simulink model "Non_isolated_SEPIC"  (R2021a)
settings: Solver=VariableStepAuto  StartTime=0.0  StopTime=0.1  RelTol=1e-3
libraries: spsSeriesRLCBranchLib x8, spsCurrentMeasurementLib x3, spsVoltageMeasurementLib x2, spsDiodeLib x1, spsMosfetLib x1, spsDCVoltageSourceLib x1, spspowerguiLib x1
settings Model: Creator=EREN-PC  LastModifiedBy=EREN-PC

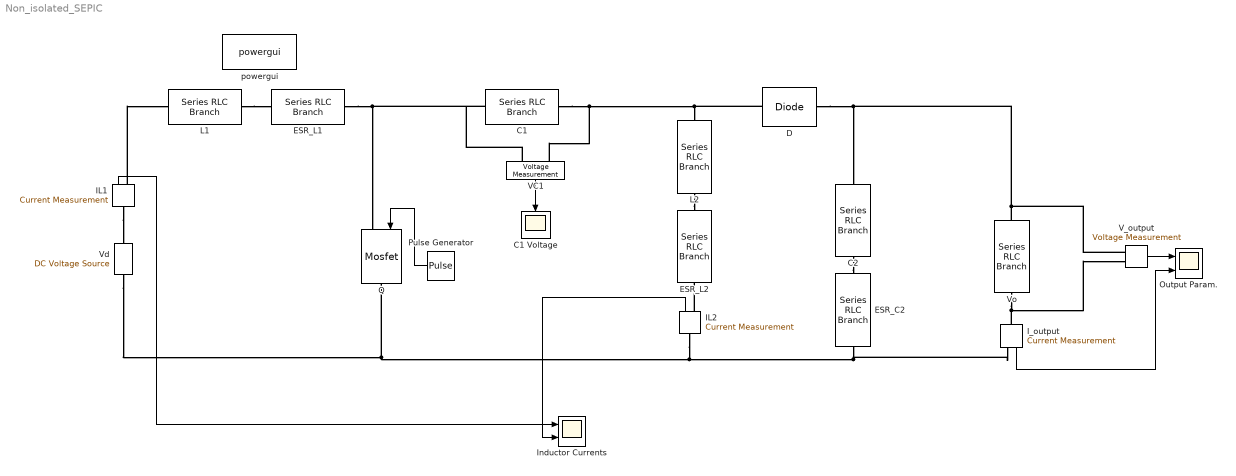
== system Non_isolated_SEPIC ==
  C1 : spsSeriesRLCBranchLib/Series RLC Branch  LConnTagsString=__new0  RConnTagsString=__new0  BranchType=C  Resistance=1  Inductance=1e-3  SetiL0=off  InitialCurrent=0  Capacitance=180e-6  Setx0=off  InitialVoltage=0  Measurements=None
  C1 Voltage : Scope
  C2 : spsSeriesRLCBranchLib/Series RLC Branch  LConnTagsString=__new0  RConnTagsString=__new0  BranchType=C  Resistance=1  Inductance=1e-3  SetiL0=off  InitialCurrent=0  Capacitance=1000e-6  Setx0=off  InitialVoltage=0  Measurements=None
  D : spsDiodeLib/Diode  Ron=0.001  Lon=0  Vf=0.420  IC=0  UseSnubber=0  Rs=500  Cs=250e-9  Measurements=off
  ESR_C2 : spsSeriesRLCBranchLib/Series RLC Branch  LConnTagsString=__new0  RConnTagsString=__new0  BranchType=R  Resistance=0.06  Inductance=1e-3  SetiL0=off  InitialCurrent=0  Capacitance=1e-6  Setx0=off  InitialVoltage=0  Measurements=None
  ESR_L1 : spsSeriesRLCBranchLib/Series RLC Branch  LConnTagsString=__new0  RConnTagsString=__new0  BranchType=R  Resistance=0.494  Inductance=1e-3  SetiL0=off  InitialCurrent=0  Capacitance=1e-6  Setx0=off  InitialVoltage=0  Measurements=None
  ESR_L2 : spsSeriesRLCBranchLib/Series RLC Branch  LConnTagsString=__new0  RConnTagsString=__new0  BranchType=R  Resistance=0.494  Inductance=1e-3  SetiL0=off  InitialCurrent=0  Capacitance=1e-6  Setx0=off  InitialVoltage=0  Measurements=None
  IL1 : spsCurrentMeasurementLib/Current Measurement  PhasorSimulation=off  OutputType=Complex  PSBequivalent=0
  IL2 : spsCurrentMeasurementLib/Current Measurement  PhasorSimulation=off  OutputType=Complex  PSBequivalent=0
  I_output : spsCurrentMeasurementLib/Current Measurement  PhasorSimulation=off  OutputType=Complex  PSBequivalent=0
  Inductor Currents : Scope  NumInputPorts=2
  L1 : spsSeriesRLCBranchLib/Series RLC Branch  LConnTagsString=__new0  RConnTagsString=__new0  BranchType=L  Resistance=1  Inductance=2.2e-3  SetiL0=off  InitialCurrent=0  Capacitance=1e-6  Setx0=off  InitialVoltage=0  Measurements=None
  L2 : spsSeriesRLCBranchLib/Series RLC Branch  LConnTagsString=__new0  RConnTagsString=__new0  BranchType=L  Resistance=1  Inductance=2.2e-3  SetiL0=off  InitialCurrent=0  Capacitance=1e-6  Setx0=off  InitialVoltage=0  Measurements=None
  Output Param. : Scope  NumInputPorts=2
  Pulse Generator : DiscretePulseGenerator  PulseType=Time based  Period=1/50000  PulseWidth=48
  Q : spsMosfetLib/Mosfet  Ron=60e-3  Lon=0  Rd=0.01  Vfd=0  IC=0  Rs=1e5  Cs=inf  Measurements=off
  VC1 : spsVoltageMeasurementLib/Voltage Measurement  PhasorSimulation=off  OutputType=Complex  PSBequivalent=0
  V_output : spsVoltageMeasurementLib/Voltage Measurement  PhasorSimulation=off  OutputType=Complex  PSBequivalent=0
  Vd : spsDCVoltageSourceLib/DC Voltage Source  Amplitude=16  Measurements=None
  Vo : spsSeriesRLCBranchLib/Series RLC Branch  LConnTagsString=__new0  RConnTagsString=__new0  BranchType=R  Resistance=6  Inductance=1e-3  SetiL0=off  InitialCurrent=0  Capacitance=1e-6  Setx0=off  InitialVoltage=0  Measurements=None
  powergui : spspowerguiLib/powergui  Priority=1  SimulationMode=Continuous  SampleTime=50e-6  frequency=60  Iterations=50  frequencyindice=0  Pbase=100e6  ErrMax=1e-4  UnitsV=kV  UnitsW=MW  buscounter=0  FunctionMessages=off  echomessages=off  EnableUseOfTLC=off  CurrentSourceSwitches=off  DisableSnubberDevices=off  DisableRonSwitches=off  DisableVfSwitches=off  DisplayEquations=off  AutomaticDiscreteSolvers=off  SolverType=Tustin/Backward Euler (TBE)  Interpol=off  ExternalGateDelay=off  methode=off  Ts=100  x0status=blocks  SPID=on  SwTol=0  HookPort=off  NonlinearTolerance=1e-4  nMaxIteration=100  ContinueOnMaxIteration=off  RestoreLinks=warning  ResistiveCurrentMeasurement=off  Frange=[0:2:500]  Ylog=off  Xlog=on  ShowGrid=off  save=off  variable=ZData  structure=0  ZoomFFT=off  StartTime=0.0  cycles=1  DisplayStyle=1  fundamental=60  FreqAxis=off  MaxFrequency=1000  frequencyindicesteady=1  RmsSteady=1  display=off
  wires:
  Pulse Generator/1 -> Q/1
  V_output/1 -> Output Param./1
  I_output/1 -> Output Param./2
  IL1/1 -> Inductor Currents/1
  IL2/1 -> Inductor Currents/2
  VC1/1 -> C1 Voltage/1
  connections:
  L1/RConn1 -- ESR_L1/LConn1
  Vo/RConn1 -- V_output/LConn2 -- I_output/LConn1
  C1/RConn1 -- VC1/LConn2 -- L2/LConn1 -- D/LConn1
  Vo/LConn1 -- C2/LConn1 -- D/RConn1 -- V_output/LConn1
  ESR_L1/RConn1 -- VC1/LConn1 -- C1/LConn1 -- Q/LConn1
  L2/RConn1 -- ESR_L2/LConn1
  C2/RConn1 -- ESR_C2/LConn1
  IL1/LConn1 -- Vd/RConn1
  IL1/RConn1 -- L1/LConn1
  Vd/LConn1 -- Q/RConn1 -- IL2/LConn1 -- I_output/RConn1 -- ESR_C2/RConn1
  IL2/RConn1 -- ESR_L2/RConn1
